simulink model "pi_send_video"  (R2016b)
settings: Solver=FixedStepAuto  StartTime=0.0  StopTime=10.0  RelTol=1e-3
libraries: embdlinuxlib x17, etargetslib x15, visionconversions x3
settings Model: SimulationMode=external  Creator=zeabus  LastModifiedBy=zeabus
settings SolverCC: PositivePriorityOrder=on
settings OptimizationCC: MaxStackSize=64
settings DebuggingCC: ParameterTunabilityLossMsg=error
settings HardwareCC: ProdBitPerPointer=32  ProdBitPerSizeT=32  ProdBitPerPtrDiffT=32  ProdLargestAtomicInteger=Long  ProdLargestAtomicFloat=Double  ProdWordSize=32  ProdHWDeviceType=ARM Compatible->ARM Cortex
settings RTWCC: SystemTargetFile=ert.tlc  HardwareBoard=Raspberry Pi  TLCOptions="-aInlineSetEventsForThisBaseRateFcn=TLC_FALSE -aSuppressMultiTaskScheduler=TLC_FALSE  -aRateBasedStepFcn=0"  TemplateMakefile=ert_default_tmf  Description=Embedded Coder  GenerateReport=on  Toolchain=GNU GCC Raspberry Pi  IncludeHyperlinkInReport=on  LaunchReport=on  GenerateTraceInfo=on  GenerateTraceReport=on  GenerateTraceReportSl=on  GenerateTraceReportSf=on  GenerateTraceReportEml=on
settings CodeAppCC: ForceParamTrailComments=on  IgnoreCustomStorageClasses=off  OperatorAnnotations=on  SimulinkDataObjDesc=on  SFDataObjDesc=on  MATLABFcnDesc=on  InsertBlockDesc=on  MATLABSourceComments=on
settings ERTTargetCC: SupportVariableSizeSignals=on

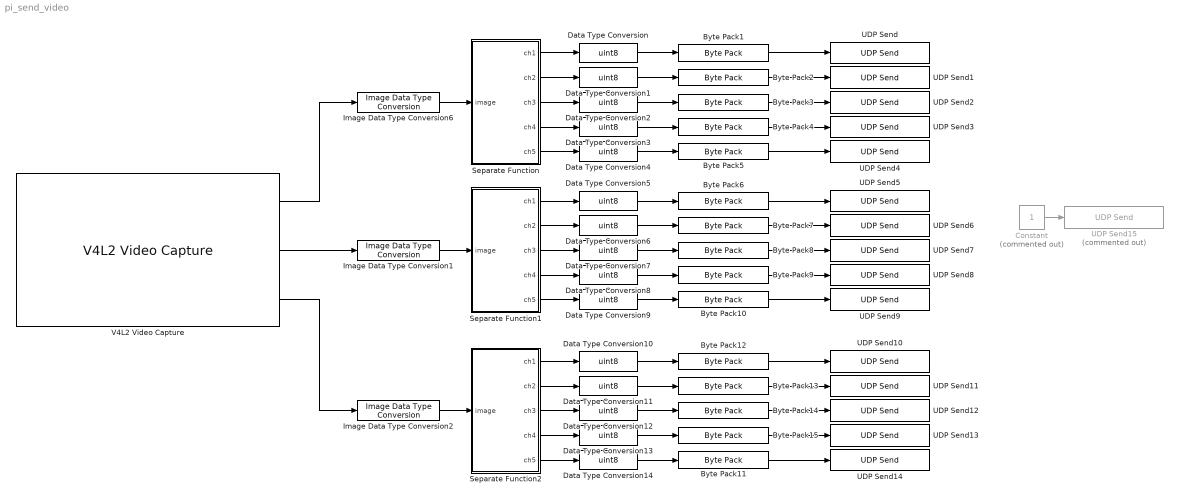
== system pi_send_video ==
  Byte Pack{1..15} (15 alike) : etargetslib/Byte Pack  datatypes={'uint8'}  byteAlign=1
  Constant : Constant  Commented=on
  Data Type Conversion{,1..14} (15 alike) : DataTypeConversion  OutDataTypeStr=uint8
  Image Data Type Conversion1 : visionconversions/Image Data Type Conversion  outDT=uint8  isSigned=on  wordLen=16  numFracBits=0
  Image Data Type Conversion2 : visionconversions/Image Data Type Conversion  outDT=uint8  isSigned=on  wordLen=16  numFracBits=0
  Image Data Type Conversion6 : visionconversions/Image Data Type Conversion  outDT=uint8  isSigned=on  wordLen=16  numFracBits=0
  Separate Function : MATLAB Function  TreatAsAtomicUnit=on
  Separate Function1 : MATLAB Function  TreatAsAtomicUnit=on
  Separate Function2 : MATLAB Function  TreatAsAtomicUnit=on
  UDP Send : embdlinuxlib/UDP Send  remoteURL='192.168.1.189'  remotePort=30000  localURL='255.255.255.255'  localPortSource=Automatically determine  localPort=-1  sampletime=-1  blockPlatform=Raspberry Pi  separateLengthPort=0
  UDP Send1 : embdlinuxlib/UDP Send  remoteURL='192.168.1.189'  remotePort=30001  localURL='255.255.255.255'  localPortSource=Automatically determine  localPort=-1  sampletime=-1  blockPlatform=Raspberry Pi  separateLengthPort=0
  UDP Send10 : embdlinuxlib/UDP Send  remoteURL='192.168.1.189'  remotePort=30010  localURL='255.255.255.255'  localPortSource=Automatically determine  localPort=-1  sampletime=-1  blockPlatform=Raspberry Pi  separateLengthPort=0
  UDP Send11 : embdlinuxlib/UDP Send  remoteURL='192.168.1.189'  remotePort=30011  localURL='255.255.255.255'  localPortSource=Automatically determine  localPort=-1  sampletime=-1  blockPlatform=Raspberry Pi  separateLengthPort=0
  UDP Send12 : embdlinuxlib/UDP Send  remoteURL='192.168.1.189'  remotePort=30012  localURL='255.255.255.255'  localPortSource=Automatically determine  localPort=-1  sampletime=-1  blockPlatform=Raspberry Pi  separateLengthPort=0
  UDP Send13 : embdlinuxlib/UDP Send  remoteURL='192.168.1.189'  remotePort=30013  localURL='255.255.255.255'  localPortSource=Automatically determine  localPort=-1  sampletime=-1  blockPlatform=Raspberry Pi  separateLengthPort=0
  UDP Send14 : embdlinuxlib/UDP Send  remoteURL='192.168.1.189'  remotePort=30014  localURL='255.255.255.255'  localPortSource=Automatically determine  localPort=-1  sampletime=-1  blockPlatform=Raspberry Pi  separateLengthPort=0
  UDP Send15 : embdlinuxlib/UDP Send  Commented=on  remoteURL='192.168.1.189'  remotePort=40000  localURL='255.255.255.255'  localPortSource=Automatically determine  localPort=-1  sampletime=-1  blockPlatform=Raspberry Pi  separateLengthPort=0
  UDP Send2 : embdlinuxlib/UDP Send  remoteURL='192.168.1.189'  remotePort=30002  localURL='255.255.255.255'  localPortSource=Automatically determine  localPort=-1  sampletime=-1  blockPlatform=Raspberry Pi  separateLengthPort=0
  UDP Send3 : embdlinuxlib/UDP Send  remoteURL='192.168.1.189'  remotePort=30003  localURL='255.255.255.255'  localPortSource=Automatically determine  localPort=-1  sampletime=-1  blockPlatform=Raspberry Pi  separateLengthPort=0
  UDP Send4 : embdlinuxlib/UDP Send  remoteURL='192.168.1.189'  remotePort=30004  localURL='255.255.255.255'  localPortSource=Automatically determine  localPort=-1  sampletime=-1  blockPlatform=Raspberry Pi  separateLengthPort=0
  UDP Send5 : embdlinuxlib/UDP Send  remoteURL='192.168.1.189'  remotePort=30005  localURL='255.255.255.255'  localPortSource=Automatically determine  localPort=-1  sampletime=-1  blockPlatform=Raspberry Pi  separateLengthPort=0
  UDP Send6 : embdlinuxlib/UDP Send  remoteURL='192.168.1.189'  remotePort=30006  localURL='255.255.255.255'  localPortSource=Automatically determine  localPort=-1  sampletime=-1  blockPlatform=Raspberry Pi  separateLengthPort=0
  UDP Send7 : embdlinuxlib/UDP Send  remoteURL='192.168.1.189'  remotePort=30007  localURL='255.255.255.255'  localPortSource=Automatically determine  localPort=-1  sampletime=-1  blockPlatform=Raspberry Pi  separateLengthPort=0
  UDP Send8 : embdlinuxlib/UDP Send  remoteURL='192.168.1.189'  remotePort=30008  localURL='255.255.255.255'  localPortSource=Automatically determine  localPort=-1  sampletime=-1  blockPlatform=Raspberry Pi  separateLengthPort=0
  UDP Send9 : embdlinuxlib/UDP Send  remoteURL='192.168.1.189'  remotePort=30009  localURL='255.255.255.255'  localPortSource=Automatically determine  localPort=-1  sampletime=-1  blockPlatform=Raspberry Pi  separateLengthPort=0
  V4L2 Video Capture : embdlinuxlib/V4L2 Video Capture  m_devName='/dev/video0'  roi=[0, 0, 640, 480]  imSizeSelection=320x240  imSize=[640, 480]  pixelFormat=RGB  pixelOrder=Planar  sampleTime=1/10  simOutput=Colorbars  blockPlatform=Raspberry Pi
  wires:
  V4L2 Video Capture/1 -> Image Data Type Conversion6/1
  V4L2 Video Capture/2 -> Image Data Type Conversion1/1
  V4L2 Video Capture/3 -> Image Data Type Conversion2/1
  Image Data Type Conversion6/1 -> Separate Function/1(image)
  Separate Function/1(ch1) -> Data Type Conversion/1
  Separate Function/2(ch2) -> Data Type Conversion1/1
  Separate Function/4(ch4) -> Data Type Conversion3/1
  Separate Function/3(ch3) -> Data Type Conversion2/1
  Separate Function/5(ch5) -> Data Type Conversion4/1
  Data Type Conversion/1 -> Byte Pack1/1
  Data Type Conversion1/1 -> Byte Pack2/1
  Data Type Conversion2/1 -> Byte Pack3/1
  Data Type Conversion3/1 -> Byte Pack4/1
  Data Type Conversion4/1 -> Byte Pack5/1
  Byte Pack1/1 -> UDP Send/1
  Byte Pack2/1 -> UDP Send1/1
  Byte Pack3/1 -> UDP Send2/1
  Byte Pack4/1 -> UDP Send3/1
  Byte Pack5/1 -> UDP Send4/1
  Image Data Type Conversion1/1 -> Separate Function1/1(image)
  Separate Function1/1(ch1) -> Data Type Conversion5/1
  Separate Function1/2(ch2) -> Data Type Conversion6/1
  Separate Function1/4(ch4) -> Data Type Conversion8/1
  Separate Function1/3(ch3) -> Data Type Conversion7/1
  Separate Function1/5(ch5) -> Data Type Conversion9/1
  Data Type Conversion5/1 -> Byte Pack6/1
  Data Type Conversion6/1 -> Byte Pack7/1
  Data Type Conversion7/1 -> Byte Pack8/1
  Data Type Conversion8/1 -> Byte Pack9/1
  Data Type Conversion9/1 -> Byte Pack10/1
  Byte Pack6/1 -> UDP Send5/1
  Byte Pack7/1 -> UDP Send6/1
  Byte Pack8/1 -> UDP Send7/1
  Byte Pack9/1 -> UDP Send8/1
  Byte Pack10/1 -> UDP Send9/1
  Image Data Type Conversion2/1 -> Separate Function2/1(image)
  Separate Function2/1(ch1) -> Data Type Conversion10/1
  Separate Function2/2(ch2) -> Data Type Conversion11/1
  Separate Function2/4(ch4) -> Data Type Conversion13/1
  Separate Function2/3(ch3) -> Data Type Conversion12/1
  Separate Function2/5(ch5) -> Data Type Conversion14/1
  Data Type Conversion10/1 -> Byte Pack12/1
  Data Type Conversion11/1 -> Byte Pack13/1
  Data Type Conversion12/1 -> Byte Pack14/1
  Data Type Conversion13/1 -> Byte Pack15/1
  Data Type Conversion14/1 -> Byte Pack11/1
  Byte Pack12/1 -> UDP Send10/1
  Byte Pack13/1 -> UDP Send11/1
  Byte Pack14/1 -> UDP Send12/1
  Byte Pack15/1 -> UDP Send13/1
  Byte Pack11/1 -> UDP Send14/1
  Constant/1 -> UDP Send15/1

== matlab function pi_send_video/Separate Function1 ==
  data: image input; ch1 output; ch2 output; ch3 output; ch4 output; ch5 output
function [ch1,ch2,ch3,ch4,ch5] = separate(image)
maxlength = 76800;
dividelength = 15360;

image = reshape(image,1,maxlength);
ch1 = image(1:dividelength);
ch2 = image(dividelength*1+1:dividelength*2);
ch3 = image(dividelength*2+1:dividelength*3);
ch4 = image(dividelength*3+1:dividelength*4);
ch5 = image(dividelength*4+1:dividelength*5);

== matlab function pi_send_video/Separate Function ==
  data: image input; ch1 output; ch2 output; ch3 output; ch4 output; ch5 output
function [ch1,ch2,ch3,ch4,ch5] = separate(image)
maxlength = 76800;
dividelength = 15360;

image = reshape(image,1,maxlength);
ch1 = image(1:dividelength);
ch2 = image(dividelength*1+1:dividelength*2);
ch3 = image(dividelength*2+1:dividelength*3);
ch4 = image(dividelength*3+1:dividelength*4);
ch5 = image(dividelength*4+1:dividelength*5);

== matlab function pi_send_video/Separate Function2 ==
  data: image input; ch1 output; ch2 output; ch3 output; ch4 output; ch5 output
function [ch1,ch2,ch3,ch4,ch5] = separate(image)
maxlength = 76800;
dividelength = 15360;

image = reshape(image,1,maxlength);
ch1 = image(1:dividelength);
ch2 = image(dividelength*1+1:dividelength*2);
ch3 = image(dividelength*2+1:dividelength*3);
ch4 = image(dividelength*3+1:dividelength*4);
ch5 = image(dividelength*4+1:dividelength*5);
